simulink model "final_version"  (R2025b)
settings: Solver=VariableStepAuto  StartTime=0.0  StopTime=10.0  RelTol=1e-3
undefined symbols (not defined in the file): entity, m, n
settings Model: Creator=39389  LastModifiedBy=39389

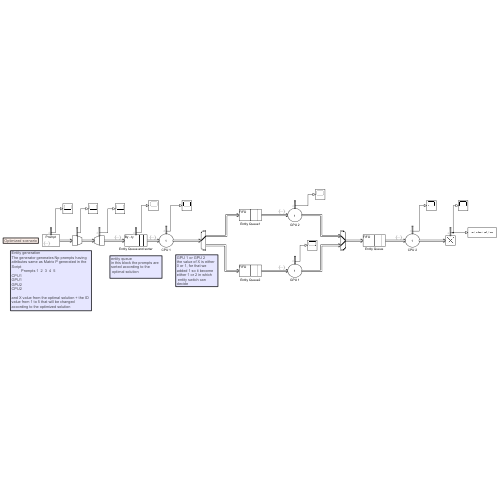
[thumbnail: Simulink's stored preview of the top-level diagram]
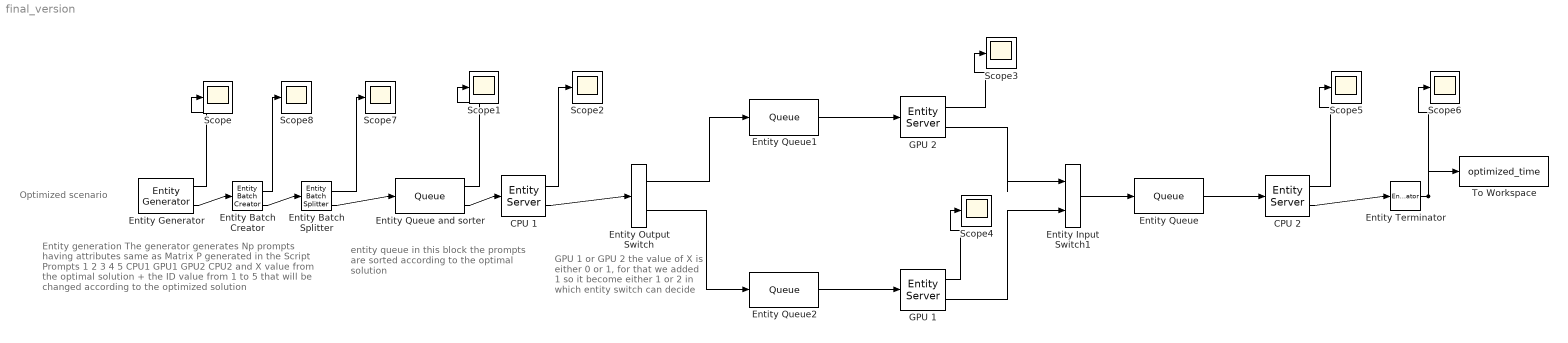
== system final_version ==
  note: Optimized scenario
  note: GPU 1 or GPU 2
      | the value of X is either
      | 0 or 1, for that we
      | added 1 so it become
      | either 1 or 2 in which
      |  entity switch can
      | decide
  note: entity queue
      | in this block the prompts are
      | sorted according to the
      |  optimal solution
  note: Entity generation
      | The generator generates Np prompts having
      | attributes same as Matrix P generated in the
      | Script
      |          Prompts 1  2  3  4  5
      | CPU1
      | GPU1
      | GPU2
      | CPU2
      |
      | and X value from the optimal solution + the ID
      | value from 1 to 5 that will be changed
      | according to the optimized solution
  CPU 1 : EntityServer  InputPortMessageModes=m  OutputPortMessageModes=n,m  Capacity=1  ServiceTimeSource=Attribute  ServiceTimeValue=CPU  ServiceTimeAttributeName=CPU1  EntryAction=|  NumberEntitiesDeparted=on
      | %disp(entity.CPU1);
      | %disp(entity.ID);
      | %disp(entity.priority)
      settings: OutputPortMap=o0,o9
  CPU 2 : EntityServer  InputPortMessageModes=m  OutputPortMessageModes=n,m  Capacity=1  ServiceTimeSource=Attribute  ServiceTimeValue=CPU  ServiceTimeAttributeName=CPU2  EntryAction=%disp(entity.CPU1)  NumberEntitiesDeparted=on
      settings: OutputPortMap=o0,o9
  Entity Input Switch1 : EntityInputSwitch  InputPortMessageModes=m,m  OutputPortMessageModes=m
  Entity Output Switch : EntityOutputSwitch  InputPortMessageModes=m  OutputPortMessageModes=m,m  SwitchingCriterion=From attribute  SwitchAttributeName=X
  Entity Batch Creator : EntityBatchCreator  InputPortMessageModes=m  OutputPortMessageModes=n,m  NumberOfEntitiesInBatch=Np  NumberOfEntitiesArrived=on
      settings: OutputPortMap=o0,o4
  Entity Batch Splitter : EntityBatchSplitter  InputPortMessageModes=m  OutputPortMessageModes=n,m  NumberOfEntitiesDeparted=on
      settings: OutputPortMap=o1,o4
  Entity Generator : EntityGenerator  OutputPortMessageModes=n,m  TimeSource=MATLAB action  IntergenerationTimeAction=|  GenerateAction=|  AttributeName=ID|CPU1|X|GPU1|GPU2|CPU2|priority  AttributeInitialValue=1|0|0|0|0|0|0  NumberEntitiesDeparted=on  EntityType=Structured  EntityTypeName=Prompt
      IntergenerationTimeAction=|
      | persistent idx itg;
      | 
      | itg = [zeros(1, N), Inf];
      | 
      | if(isempty(idx))
      |     idx = 1;
      |     dt = itg(idx);
      |     idx = idx + 1;
      | end
      | 
      | dt = itg(idx);
      | idx = idx + 1;
      GenerateAction=|
      | entity.ID=mod(entitySys.id,Np+1);
      | entity.CPU1=P(1,entity.ID);
      | entity.GPU1=P(2,entity.ID);
      | entity.GPU2=P(3,entity.ID);
      | entity.CPU2=P(4,entity.ID);
      | entity.X=x_opt(entity.ID)+1;
      | %priority_map = [0 0 0 0 0];  % initialize
      | %for k = 1:length(cpu1_sequence)
      | %    priority_map(cpu1_sequence(k)) = k;
      | %end
      | 
      | entity.priority = priority_map(entity.ID);
      | %disp(entity.priority)
      | %disp(entity.ID)
      settings: OutputPortMap=o0,o3
  Entity Queue : Queue  InputPortMessageModes=m  OutputPortMessageModes=m
  Entity Queue and sorter : Queue  InputPortMessageModes=m  OutputPortMessageModes=n,m  QueueType=Priority  PrioritySource=priority  EntryAction=|  NumberEntitiesDeparted=on
      | %disp(entity.ID)
      | %disp(entity.priority)
      | %priority_map = [0 0 0 0 0];  % initialize
      | %for k = 1:length(cpu1_sequence)
      | %    priority_map(cpu1_sequence(k)) = k;
      | %end
      | 
      | %entity.priority = priority_map(entity.ID);
      | %disp(entity.priority)
      | %disp(entity.ID)
      settings: OutputPortMap=o0,o5
  Entity Queue1 : Queue  InputPortMessageModes=m  OutputPortMessageModes=m
  Entity Queue2 : Queue  InputPortMessageModes=m  OutputPortMessageModes=m
  Entity Terminator : EntityTerminator  InputPortMessageModes=m  NumberEntitiesArrived=on
      settings: OutputPortMap=o0
  GPU 1 : EntityServer  InputPortMessageModes=m  OutputPortMessageModes=n,m  Capacity=1  ServiceTimeSource=Attribute  ServiceTimeValue=CPU  ServiceTimeAttributeName=GPU1  EntryAction=%disp(entity.CPU1)  NumberEntitiesDeparted=on
      settings: OutputPortMap=o0,o9
  GPU 2 : EntityServer  InputPortMessageModes=m  OutputPortMessageModes=n,m  Capacity=1  ServiceTimeSource=Attribute  ServiceTimeValue=CPU  ServiceTimeAttributeName=GPU2  EntryAction=%disp(entity.CPU1)  NumberEntitiesDeparted=on
      settings: OutputPortMap=o0,o9
  Scope{,1..8} (9 alike) : Scope
      Scope settings: ActiveDisplayYMinimum=-1  ActiveDisplayYMaximum=1
      Scope1 settings: ActiveDisplayYMinimum=0.057553101027644882  ActiveDisplayYMaximum=5.8456781010276444
      Scope2 settings: ActiveDisplayYMinimum=-1  ActiveDisplayYMaximum=1  DataLoggingVariableName=ScopeData2
      Scope3 settings: ActiveDisplayYMinimum=-1  ActiveDisplayYMaximum=1  DataLoggingVariableName=ScopeData3
      Scope4 settings: ActiveDisplayYMinimum=-1  ActiveDisplayYMaximum=1  DataLoggingVariableName=ScopeData4
      Scope5 settings: ActiveDisplayYMinimum=-1  ActiveDisplayYMaximum=1  DataLoggingVariableName=ScopeData5
      Scope6 settings: ActiveDisplayYMinimum=0.20590799746406982  ActiveDisplayYMaximum=1.5385984843033593  DataLoggingVariableName=ScopeData6
      Scope7 settings: ActiveDisplayYMinimum=-1  ActiveDisplayYMaximum=1  DataLoggingVariableName=ScopeData7
      Scope8 settings: ActiveDisplayYMinimum=-1  ActiveDisplayYMaximum=1  DataLoggingVariableName=ScopeData8
  To Workspace : ToWorkspace  VariableName=optimized_time  SaveFormat=Timeseries  SampleTime=-1
  wires:
  Entity Queue and sorter/2 -> CPU 1/1
  Entity Queue and sorter/1 -> Scope1/1
  Entity Generator/1 -> Scope/1
  CPU 1/1 -> Scope2/1
  CPU 1/2 -> Entity Output Switch/1
  Entity Output Switch/1 -> Entity Queue1/1
  Entity Output Switch/2 -> Entity Queue2/1
  Entity Queue1/1 -> GPU 2/1
  Entity Queue2/1 -> GPU 1/1
  GPU 2/2 -> Entity Input Switch1/1
  GPU 1/2 -> Entity Input Switch1/2
  Entity Input Switch1/1 -> Entity Queue/1
  Entity Queue/1 -> CPU 2/1
  CPU 2/2 -> Entity Terminator/1
  GPU 2/1 -> Scope3/1
  GPU 1/1 -> Scope4/1
  CPU 2/1 -> Scope5/1
  Entity Terminator/1 -> Scope6/1, To Workspace/1
  Entity Generator/2 -> Entity Batch Creator/1
  Entity Batch Creator/2 -> Entity Batch Splitter/1
  Entity Batch Splitter/2 -> Entity Queue and sorter/1
  Entity Batch Splitter/1 -> Scope7/1
  Entity Batch Creator/1 -> Scope8/1
